simulink model "walkingRobot_stable"  (R2020a)
settings: Solver=ode15s  StartTime=0.0  StopTime=10  EnableMultiTasking=on
PreLoadFcn:
  | robotParameters
  | load('defaultsimulationinputs.mat')
values from neighbouring files (symbols this model uses):
  init_angs_L = zeros(6,1)    [robotParameters.m]
  init_angs_R = zeros(6,1)    [robotParameters.m]
  motion_time_constant = 0.001    [robotParameters.m]
libraries: simulink_extras x12, walkingRobotUtils x3, simulink x1
settings Model: SimulationMode=accelerator  Creator=bkim  LastModifiedBy=nikhil
settings DataIOCC: ReturnWorkspaceOutputs=off  OutputSaveName=simout  OutputTimes=0:0.01:10
settings OptimizationCC: LifeSpan=inf
settings DebuggingCC: AllowSymbolicDim=off  PregeneratedLibrarySubsystemCodeDiagnostic=none  SFUnexpectedBacktrackingDiag=warning  SFNoUnconditionalDefaultTransitionDiag=warning  SFExecutionAtInitializationDiag=none  UnitsInconsistencyMsg=none  ArithmeticOperatorsInVariantConditions=warning
settings SFSimCC: SimUseLocalCustomCode=off  CustomCodeUndefinedFunction=UseInterfaceOnly
settings RTWCC: RTWUseLocalCustomCode=off
settings CodeAppCC: StateflowObjectComments=on
settings GRTTargetCC: TargetLangStandard=C89/C90 (ANSI)
settings ConfigComp: CovMetricSettings=dw  CovHtmlReporting=on  CovSaveCumulativeToWorkspaceVar=on  CovSaveSingleToWorkspaceVar=on  CovExternalEMLEnable=off  CovSFcnEnable=off
settings SimscapeCC: SimscapeNormalizeSystem=off  SimscapeLogOpenViewer=on  SimscapeLogLimitData=off  SimscapeLogDataHistory=10000
settings ConfigurationSet: Description=SimMechanics 2G
settings DiagnosticsConfigSet: SimMechanicsRigidlyBoundBlock=none
settings ExplorerConfigSet: InternalSimMechanicsExplorerSettings="<ExplorerConfiguration><canonicalview>default</canonicalview><AnimationSetting><BasePlaybackSpeed>1.0</BasePlaybackSpeed><PlaybackSpeedFactor>1.0</PlaybackSpeedFactor></AnimationSetting><TilePanel><TileInfo><Tiles Columns=\"1\" Count=\"1\" Rows=\"1\"><Column Weight=\"1\"/><Row Weight=\"1\"/><Tile Height=\"1\" Width=\"1\" X=\"0\" Y=\"0\"/></Tiles></TileInfo><SceneInfo><SceneViewer><BGColor><R>0.60000002384185791</R><G>0.60000002384185791</G><B>0.60000002384185791</B></BGColor><Camera><DoPerspective>off</DoPerspective><Position><X>-7.90762128242833562</X><Y>23.8081096481694914</Y><Z>5.91146841204722939</Z></Position><Center><X>-0.406277996262525587</X><Y>0.615564294304502546</Y><Z>-0.277309600720595628</Z></Center><Up><X>0.182671955115720652</X><Y>-0.197900690545468771</Y><Z>0.963050504125213092</Z></Up><ViewLimDist>1</ViewLimDist><YLim>2.56954837368236522</YLim><XLim>3.29520786810192234</XLim></Camera></SceneViewer></SceneInfo></TilePanel><MechEditorPanel><Cameras/><GfxPanelCameraMap/><VideoCreator><PlaybackSpeedRatio>1.0</PlaybackSpeedRatio><FrameRate>30</FrameRate><VideoFormat>Motion JPEG AVI</VideoFormat><FrameSize>auto</FrameSize></VideoCreator></MechEditorPanel></ExplorerConfiguration>"

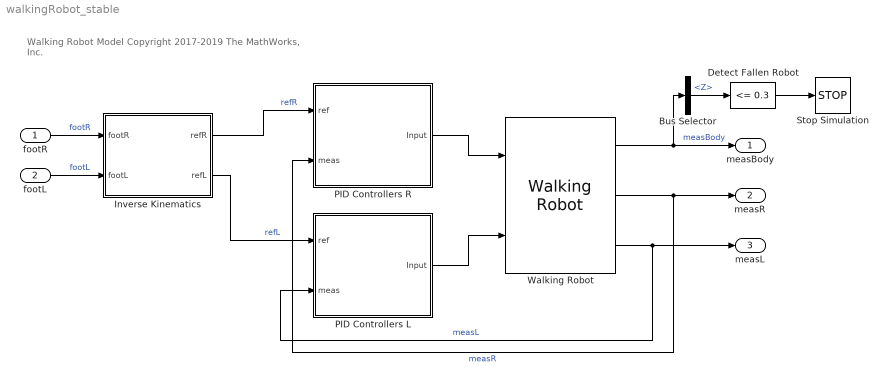
== system walkingRobot_stable ==
  note: Walking Robot Model
      |
      | Copyright 2017-2019 The MathWorks, Inc.
  footR : Inport
  footL : Inport  Port=2
  Bus Selector : BusSelector  OutputSignals=Z
  Detect Fallen Robot : simulink/Logic and Bit Operations/Compare To Constant  relop=<=  const=0.3  OutDataTypeStr=boolean
  Inverse Kinematics : Subsystem
  PID Controllers L : Subsystem
  PID Controllers R : Subsystem
  Stop Simulation : Stop
  Walking Robot : walkingRobotUtils/Walking Robot  SystemSampleTime=-1  Latency=0  AutoFrameSizeCalculation=off
  measBody : Outport  VectorParamsAs1DForOutWhenUnconnected=off
  measR : Outport  Port=2  VectorParamsAs1DForOutWhenUnconnected=off
  measL : Outport  Port=3  VectorParamsAs1DForOutWhenUnconnected=off
  wires:
  Walking Robot/3 -> PID Controllers L/2(meas), measL/1  "measL"
  Walking Robot/2 -> PID Controllers R/2(meas), measR/1  "measR"
  PID Controllers R/1(Input) -> Walking Robot/1
  PID Controllers L/1(Input) -> Walking Robot/2
  footR/1 -> Inverse Kinematics/1(footR)  "footR"
  footL/1 -> Inverse Kinematics/2(footL)  "footL"
  Walking Robot/1 -> Bus Selector/1, measBody/1  "measBody"
  Bus Selector/1 -> Detect Fallen Robot/1  "<Z>"
  Detect Fallen Robot/1 -> Stop Simulation/1
  Inverse Kinematics/1(refR) -> PID Controllers R/1(ref)  "refR"
  Inverse Kinematics/2(refL) -> PID Controllers L/1(ref)  "refL"

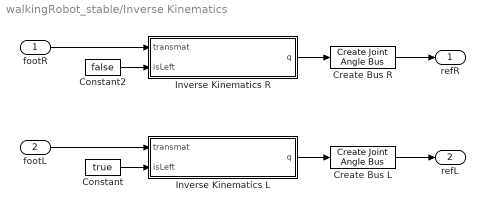
== system walkingRobot_stable/Inverse Kinematics ==
  footR : Inport
  footL : Inport  Port=2
  Constant : Constant  Value=true
  Constant2 : Constant  Value=false
  Create Bus L : walkingRobotUtils/Create Joint Angle Bus  SystemSampleTime=-1  Latency=0  AutoFrameSizeCalculation=off
  Create Bus R : walkingRobotUtils/Create Joint Angle Bus  SystemSampleTime=-1  Latency=0  AutoFrameSizeCalculation=off
  Inverse Kinematics L : MATLAB Function  TreatAsAtomicUnit=on
  Inverse Kinematics R : MATLAB Function  TreatAsAtomicUnit=on
  refR : Outport
  refL : Outport  Port=2
  wires:
  footR/1 -> Inverse Kinematics R/1(transmat)
  Inverse Kinematics L/1(q) -> Create Bus L/1
  Constant2/1 -> Inverse Kinematics R/2(isLeft)
  Create Bus R/1 -> refR/1
  Create Bus L/1 -> refL/1
  Constant/1 -> Inverse Kinematics L/2(isLeft)
  Inverse Kinematics R/1(q) -> Create Bus R/1
  footL/1 -> Inverse Kinematics L/1(transmat)

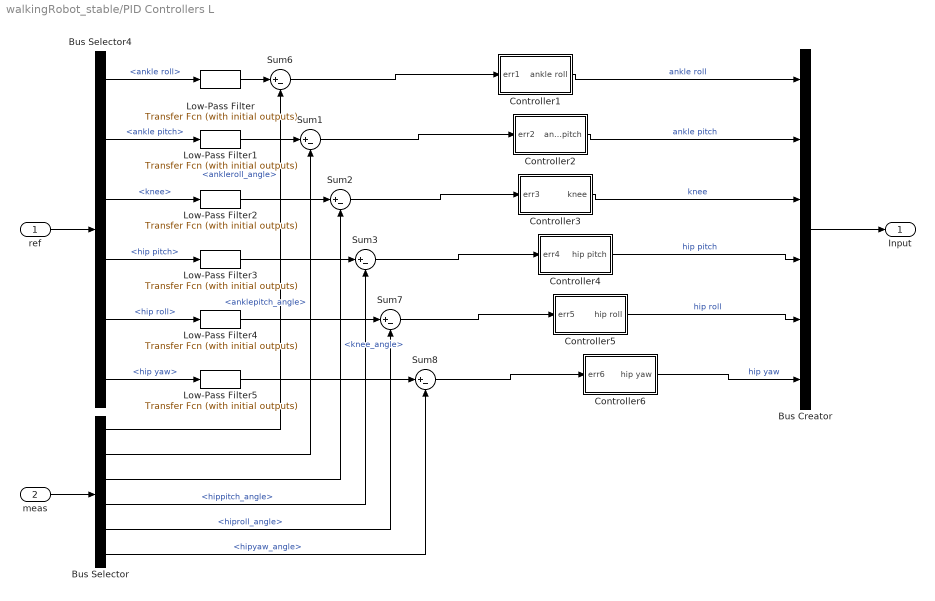
== system walkingRobot_stable/PID Controllers L ==
  ref : Inport
  meas : Inport  Port=2
  Bus Creator : BusCreator  Inputs=6
  Bus Selector : BusSelector  OutputSignals=ankleroll_angle,anklepitch_angle,knee_angle,hippitch_angle,hiproll_angle,hipyaw_angle
  Bus Selector4 : BusSelector  OutputSignals=ankle roll,ankle pitch,knee,hip pitch,hip roll,hip yaw
  Controller1 : Subsystem
  Controller2 : Subsystem
  Controller3 : Subsystem
  Controller4 : Subsystem
  Controller5 : Subsystem
  Controller6 : Subsystem
  Low-Pass Filter : simulink_extras/Additional Linear/Transfer Fcn (with initial outputs)  N=[(1/motion_time_constant)^2]  D=[1 2/motion_time_constant (1/motion_time_constant)^2]  Y0=init_angs_L(6)  U0=init_angs_L(6)
  Low-Pass Filter1 : simulink_extras/Additional Linear/Transfer Fcn (with initial outputs)  N=[(1/motion_time_constant)^2]  D=[1 2/motion_time_constant (1/motion_time_constant)^2]  Y0=init_angs_L(5)  U0=init_angs_L(5)
  Low-Pass Filter2 : simulink_extras/Additional Linear/Transfer Fcn (with initial outputs)  N=[(1/motion_time_constant)^2]  D=[1 2/motion_time_constant (1/motion_time_constant)^2]  Y0=init_angs_L(4)  U0=init_angs_L(4)
  Low-Pass Filter3 : simulink_extras/Additional Linear/Transfer Fcn (with initial outputs)  N=[(1/motion_time_constant)^2]  D=[1 2/motion_time_constant (1/motion_time_constant)^2]  Y0=init_angs_L(3)  U0=init_angs_L(3)
  Low-Pass Filter4 : simulink_extras/Additional Linear/Transfer Fcn (with initial outputs)  N=[(1/motion_time_constant)^2]  D=[1 2/motion_time_constant (1/motion_time_constant)^2]  Y0=init_angs_L(2)  U0=init_angs_L(2)
  Low-Pass Filter5 : simulink_extras/Additional Linear/Transfer Fcn (with initial outputs)  N=[(1/motion_time_constant)^2]  D=[1 2/motion_time_constant (1/motion_time_constant)^2]  Y0=init_angs_L(1)  U0=init_angs_L(1)
  Sum{1..3,6..8} (6 alike) : Sum  Inputs=|+-
  Input : Outport  VectorParamsAs1DForOutWhenUnconnected=off
  wires:
  Low-Pass Filter5/1 -> Sum8/1
  Low-Pass Filter/1 -> Sum6/1
  Bus Selector4/6 -> Low-Pass Filter5/1  "<hip yaw>"
  Bus Selector4/2 -> Low-Pass Filter1/1  "<ankle pitch>"
  Bus Selector4/4 -> Low-Pass Filter3/1  "<hip pitch>"
  Controller6/1(hip yaw) -> Bus Creator/6  "hip yaw"
  Bus Selector4/3 -> Low-Pass Filter2/1  "<knee>"
  Bus Selector4/1 -> Low-Pass Filter/1  "<ankle roll>"
  Bus Selector/3 -> Sum2/2  "<knee_angle>"
  Bus Selector4/5 -> Low-Pass Filter4/1  "<hip roll>"
  ref/1 -> Bus Selector4/1
  Low-Pass Filter3/1 -> Sum3/1
  Bus Selector/6 -> Sum8/2  "<hipyaw_angle>"
  Bus Selector/5 -> Sum7/2  "<hiproll_angle>"
  Low-Pass Filter1/1 -> Sum1/1
  Bus Creator/1 -> Input/1
  Bus Selector/1 -> Sum6/2  "<ankleroll_angle>"
  Low-Pass Filter2/1 -> Sum2/1
  Low-Pass Filter4/1 -> Sum7/1
  Bus Selector/4 -> Sum3/2  "<hippitch_angle>"
  Bus Selector/2 -> Sum1/2  "<anklepitch_angle>"
  meas/1 -> Bus Selector/1
  Controller1/1(ankle roll) -> Bus Creator/1  "ankle roll"
  Sum7/1 -> Controller5/1(err5)
  Sum6/1 -> Controller1/1(err1)
  Controller3/1(knee) -> Bus Creator/3  "knee"
  Sum1/1 -> Controller2/1(err2)
  Controller4/1(hip pitch) -> Bus Creator/4  "hip pitch"
  Sum2/1 -> Controller3/1(err3)
  Sum8/1 -> Controller6/1(err6)
  Sum3/1 -> Controller4/1(err4)
  Controller5/1(hip roll) -> Bus Creator/5  "hip roll"
  Controller2/1(ankle pitch) -> Bus Creator/2  "ankle pitch"

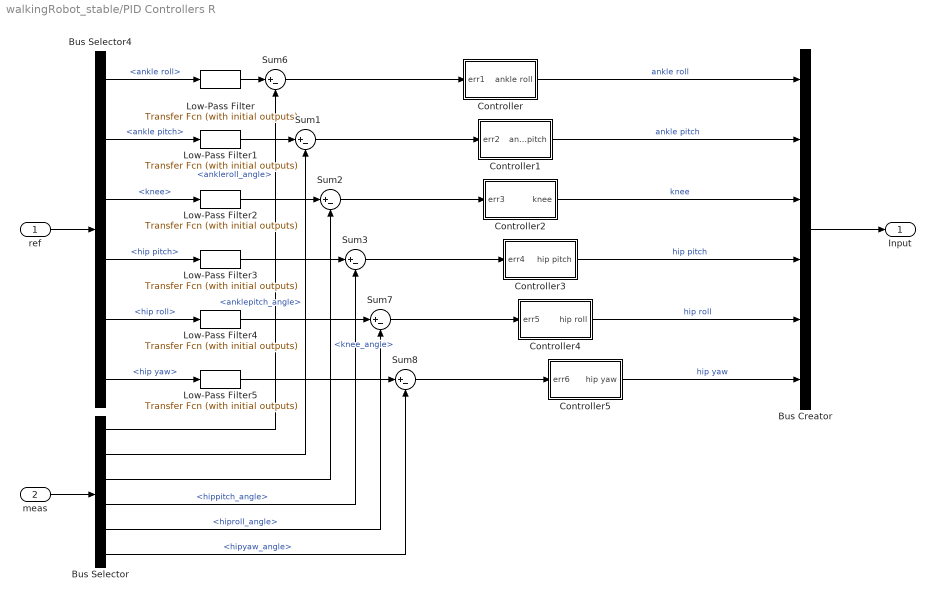
== system walkingRobot_stable/PID Controllers R ==
  ref : Inport
  meas : Inport  Port=2
  Bus Creator : BusCreator  Inputs=6
  Bus Selector : BusSelector  OutputSignals=ankleroll_angle,anklepitch_angle,knee_angle,hippitch_angle,hiproll_angle,hipyaw_angle
  Bus Selector4 : BusSelector  OutputSignals=ankle roll,ankle pitch,knee,hip pitch,hip roll,hip yaw
  Controller : Subsystem
  Controller1 : Subsystem
  Controller2 : Subsystem
  Controller3 : Subsystem
  Controller4 : Subsystem
  Controller5 : Subsystem
  Low-Pass Filter : simulink_extras/Additional Linear/Transfer Fcn (with initial outputs)  N=[(1/motion_time_constant)^2]  D=[1 2/motion_time_constant (1/motion_time_constant)^2]  Y0=init_angs_R(6)  U0=init_angs_R(6)
  Low-Pass Filter1 : simulink_extras/Additional Linear/Transfer Fcn (with initial outputs)  N=[(1/motion_time_constant)^2]  D=[1 2/motion_time_constant (1/motion_time_constant)^2]  Y0=init_angs_R(5)  U0=init_angs_R(5)
  Low-Pass Filter2 : simulink_extras/Additional Linear/Transfer Fcn (with initial outputs)  N=[(1/motion_time_constant)^2]  D=[1 2/motion_time_constant (1/motion_time_constant)^2]  Y0=init_angs_R(4)  U0=init_angs_R(4)
  Low-Pass Filter3 : simulink_extras/Additional Linear/Transfer Fcn (with initial outputs)  N=[(1/motion_time_constant)^2]  D=[1 2/motion_time_constant (1/motion_time_constant)^2]  Y0=init_angs_R(3)  U0=init_angs_R(3)
  Low-Pass Filter4 : simulink_extras/Additional Linear/Transfer Fcn (with initial outputs)  N=[(1/motion_time_constant)^2]  D=[1 2/motion_time_constant (1/motion_time_constant)^2]  Y0=init_angs_R(2)  U0=init_angs_R(2)
  Low-Pass Filter5 : simulink_extras/Additional Linear/Transfer Fcn (with initial outputs)  N=[(1/motion_time_constant)^2]  D=[1 2/motion_time_constant (1/motion_time_constant)^2]  Y0=init_angs_R(1)  U0=init_angs_R(1)
  Sum{1..3,6..8} (6 alike) : Sum  Inputs=|+-
  Input : Outport  VectorParamsAs1DForOutWhenUnconnected=off
  wires:
  meas/1 -> Bus Selector/1
  Bus Selector/2 -> Sum1/2  "<anklepitch_angle>"
  Bus Selector/4 -> Sum3/2  "<hippitch_angle>"
  Low-Pass Filter4/1 -> Sum7/1
  Low-Pass Filter2/1 -> Sum2/1
  Sum8/1 -> Controller5/1(err6)
  Bus Selector/1 -> Sum6/2  "<ankleroll_angle>"
  Bus Creator/1 -> Input/1
  Low-Pass Filter1/1 -> Sum1/1
  Bus Selector/5 -> Sum7/2  "<hiproll_angle>"
  Controller3/1(hip pitch) -> Bus Creator/4  "hip pitch"
  Bus Selector/6 -> Sum8/2  "<hipyaw_angle>"
  Low-Pass Filter3/1 -> Sum3/1
  Controller/1(ankle roll) -> Bus Creator/1  "ankle roll"
  Sum1/1 -> Controller1/1(err2)
  Sum2/1 -> Controller2/1(err3)
  ref/1 -> Bus Selector4/1
  Sum3/1 -> Controller3/1(err4)
  Bus Selector4/5 -> Low-Pass Filter4/1  "<hip roll>"
  Sum7/1 -> Controller4/1(err5)
  Bus Selector/3 -> Sum2/2  "<knee_angle>"
  Sum6/1 -> Controller/1(err1)
  Bus Selector4/1 -> Low-Pass Filter/1  "<ankle roll>"
  Bus Selector4/3 -> Low-Pass Filter2/1  "<knee>"
  Controller2/1(knee) -> Bus Creator/3  "knee"
  Controller5/1(hip yaw) -> Bus Creator/6  "hip yaw"
  Controller1/1(ankle pitch) -> Bus Creator/2  "ankle pitch"
  Bus Selector4/4 -> Low-Pass Filter3/1  "<hip pitch>"
  Bus Selector4/2 -> Low-Pass Filter1/1  "<ankle pitch>"
  Controller4/1(hip roll) -> Bus Creator/5  "hip roll"
  Bus Selector4/6 -> Low-Pass Filter5/1  "<hip yaw>"
  Low-Pass Filter/1 -> Sum6/1
  Low-Pass Filter5/1 -> Sum8/1

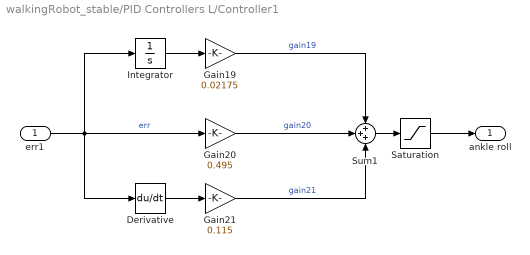
== system walkingRobot_stable/PID Controllers L/Controller1 ==
  err1 : Inport
  Derivative : Derivative
  Gain19 : Gain  Gain=0.02175
  Gain20 : Gain  Gain=0.495
  Gain21 : Gain  Gain=0.115
  Integrator : Integrator
  Saturation : Saturate  UpperLimit=15  LowerLimit=-15
  Sum1 : Sum  Inputs=+++
  ankle roll : Outport
  wires:
  Gain19/1 -> Sum1/1  "gain19"
  Saturation/1 -> ankle roll/1
  Gain20/1 -> Sum1/2  "gain20"
  Gain21/1 -> Sum1/3  "gain21"
  err1/1 -> Derivative/1, Gain20/1, Integrator/1  "err"
  Derivative/1 -> Gain21/1
  Sum1/1 -> Saturation/1
  Integrator/1 -> Gain19/1

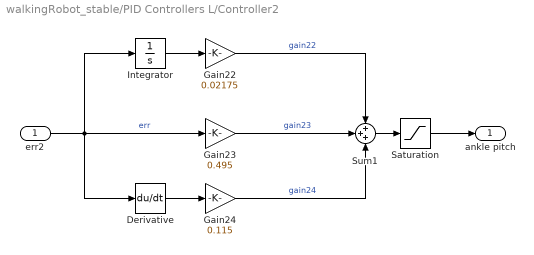
== system walkingRobot_stable/PID Controllers L/Controller2 ==
  err2 : Inport
  Derivative : Derivative
  Gain22 : Gain  Gain=0.02175
  Gain23 : Gain  Gain=0.495
  Gain24 : Gain  Gain=0.115
  Integrator : Integrator
  Saturation : Saturate  UpperLimit=15  LowerLimit=-15
  Sum1 : Sum  Inputs=+++
  ankle pitch : Outport
  wires:
  Gain22/1 -> Sum1/1  "gain22"
  Saturation/1 -> ankle pitch/1
  Gain23/1 -> Sum1/2  "gain23"
  Gain24/1 -> Sum1/3  "gain24"
  err2/1 -> Derivative/1, Gain23/1, Integrator/1  "err"
  Derivative/1 -> Gain24/1
  Sum1/1 -> Saturation/1
  Integrator/1 -> Gain22/1

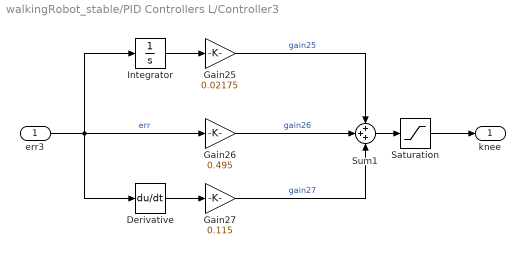
== system walkingRobot_stable/PID Controllers L/Controller3 ==
  err3 : Inport
  Derivative : Derivative
  Gain25 : Gain  Gain=0.02175
  Gain26 : Gain  Gain=0.495
  Gain27 : Gain  Gain=0.115
  Integrator : Integrator
  Saturation : Saturate  UpperLimit=15  LowerLimit=-15
  Sum1 : Sum  Inputs=+++
  knee : Outport
  wires:
  Gain25/1 -> Sum1/1  "gain25"
  Saturation/1 -> knee/1
  Gain26/1 -> Sum1/2  "gain26"
  Gain27/1 -> Sum1/3  "gain27"
  err3/1 -> Derivative/1, Gain26/1, Integrator/1  "err"
  Derivative/1 -> Gain27/1
  Sum1/1 -> Saturation/1
  Integrator/1 -> Gain25/1

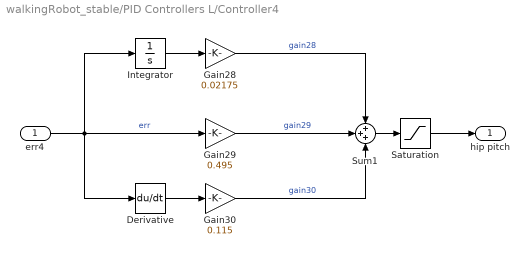
== system walkingRobot_stable/PID Controllers L/Controller4 ==
  err4 : Inport
  Derivative : Derivative
  Gain28 : Gain  Gain=0.02175
  Gain29 : Gain  Gain=0.495
  Gain30 : Gain  Gain=0.115
  Integrator : Integrator
  Saturation : Saturate  UpperLimit=15  LowerLimit=-15
  Sum1 : Sum  Inputs=+++
  hip pitch : Outport
  wires:
  Gain28/1 -> Sum1/1  "gain28"
  Saturation/1 -> hip pitch/1
  Gain29/1 -> Sum1/2  "gain29"
  Gain30/1 -> Sum1/3  "gain30"
  err4/1 -> Derivative/1, Gain29/1, Integrator/1  "err"
  Derivative/1 -> Gain30/1
  Sum1/1 -> Saturation/1
  Integrator/1 -> Gain28/1

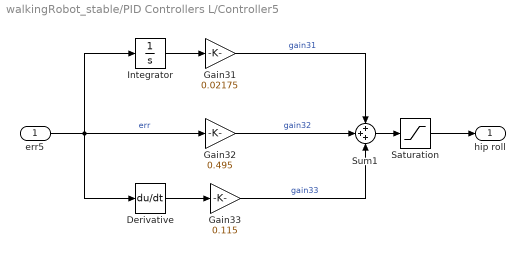
== system walkingRobot_stable/PID Controllers L/Controller5 ==
  err5 : Inport
  Derivative : Derivative
  Gain31 : Gain  Gain=0.02175
  Gain32 : Gain  Gain=0.495
  Gain33 : Gain  Gain=0.115
  Integrator : Integrator
  Saturation : Saturate  UpperLimit=15  LowerLimit=-15
  Sum1 : Sum  Inputs=+++
  hip roll : Outport
  wires:
  Gain31/1 -> Sum1/1  "gain31"
  Saturation/1 -> hip roll/1
  Gain32/1 -> Sum1/2  "gain32"
  Gain33/1 -> Sum1/3  "gain33"
  err5/1 -> Derivative/1, Gain32/1, Integrator/1  "err"
  Derivative/1 -> Gain33/1
  Sum1/1 -> Saturation/1
  Integrator/1 -> Gain31/1

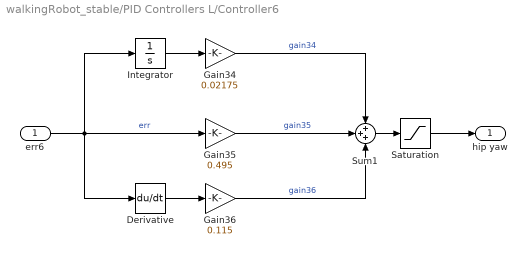
== system walkingRobot_stable/PID Controllers L/Controller6 ==
  err6 : Inport
  Derivative : Derivative
  Gain34 : Gain  Gain=0.02175
  Gain35 : Gain  Gain=0.495
  Gain36 : Gain  Gain=0.115
  Integrator : Integrator
  Saturation : Saturate  UpperLimit=15  LowerLimit=-15
  Sum1 : Sum  Inputs=+++
  hip yaw : Outport
  wires:
  Gain34/1 -> Sum1/1  "gain34"
  Saturation/1 -> hip yaw/1
  Gain35/1 -> Sum1/2  "gain35"
  Gain36/1 -> Sum1/3  "gain36"
  err6/1 -> Derivative/1, Gain35/1, Integrator/1  "err"
  Derivative/1 -> Gain36/1
  Sum1/1 -> Saturation/1
  Integrator/1 -> Gain34/1

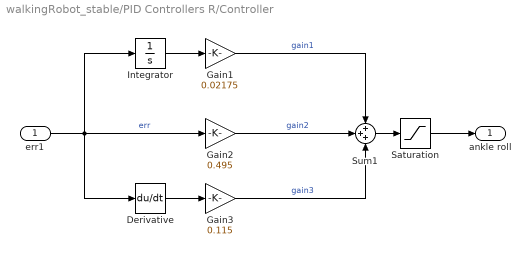
== system walkingRobot_stable/PID Controllers R/Controller ==
  err1 : Inport
  Derivative : Derivative
  Gain1 : Gain  Gain=0.02175
  Gain2 : Gain  Gain=0.495
  Gain3 : Gain  Gain=0.115
  Integrator : Integrator
  Saturation : Saturate  UpperLimit=15  LowerLimit=-15
  Sum1 : Sum  Inputs=+++
  ankle roll : Outport
  wires:
  Gain1/1 -> Sum1/1  "gain1"
  Saturation/1 -> ankle roll/1
  Gain2/1 -> Sum1/2  "gain2"
  Gain3/1 -> Sum1/3  "gain3"
  err1/1 -> Derivative/1, Gain2/1, Integrator/1  "err"
  Derivative/1 -> Gain3/1
  Sum1/1 -> Saturation/1
  Integrator/1 -> Gain1/1

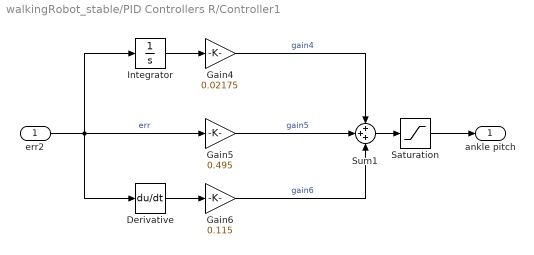
== system walkingRobot_stable/PID Controllers R/Controller1 ==
  err2 : Inport
  Derivative : Derivative
  Gain4 : Gain  Gain=0.02175
  Gain5 : Gain  Gain=0.495
  Gain6 : Gain  Gain=0.115
  Integrator : Integrator
  Saturation : Saturate  UpperLimit=15  LowerLimit=-15
  Sum1 : Sum  Inputs=+++
  ankle pitch : Outport
  wires:
  Gain4/1 -> Sum1/1  "gain4"
  Saturation/1 -> ankle pitch/1
  Gain5/1 -> Sum1/2  "gain5"
  Gain6/1 -> Sum1/3  "gain6"
  err2/1 -> Derivative/1, Gain5/1, Integrator/1  "err"
  Derivative/1 -> Gain6/1
  Sum1/1 -> Saturation/1
  Integrator/1 -> Gain4/1

== system walkingRobot_stable/PID Controllers R/Controller2 ==
  err3 : Inport
  Derivative : Derivative
  Gain7 : Gain  Gain=0.02175
  Gain8 : Gain  Gain=0.495
  Gain9 : Gain  Gain=0.115
  Integrator : Integrator
  Saturation : Saturate  UpperLimit=15  LowerLimit=-15
  Sum1 : Sum  Inputs=+++
  knee : Outport
  wires:
  Gain7/1 -> Sum1/1  "gain7"
  Saturation/1 -> knee/1
  Gain8/1 -> Sum1/2  "gain8"
  Gain9/1 -> Sum1/3  "gain9"
  err3/1 -> Derivative/1, Gain8/1, Integrator/1  "err"
  Derivative/1 -> Gain9/1
  Sum1/1 -> Saturation/1
  Integrator/1 -> Gain7/1

== system walkingRobot_stable/PID Controllers R/Controller3 ==
  err4 : Inport
  Derivative : Derivative
  Gain10 : Gain  Gain=0.02175
  Gain11 : Gain  Gain=0.495
  Gain12 : Gain  Gain=0.115
  Integrator : Integrator
  Saturation : Saturate  UpperLimit=15  LowerLimit=-15
  Sum1 : Sum  Inputs=+++
  hip pitch : Outport
  wires:
  Gain10/1 -> Sum1/1  "gain10"
  Saturation/1 -> hip pitch/1
  Gain11/1 -> Sum1/2  "gain11"
  Gain12/1 -> Sum1/3  "gain12"
  err4/1 -> Derivative/1, Gain11/1, Integrator/1  "err"
  Derivative/1 -> Gain12/1
  Sum1/1 -> Saturation/1
  Integrator/1 -> Gain10/1

== system walkingRobot_stable/PID Controllers R/Controller4 ==
  err5 : Inport
  Derivative : Derivative
  Gain13 : Gain  Gain=0.02175
  Gain14 : Gain  Gain=0.495
  Gain15 : Gain  Gain=0.115
  Integrator : Integrator
  Saturation : Saturate  UpperLimit=15  LowerLimit=-15
  Sum1 : Sum  Inputs=+++
  hip roll : Outport
  wires:
  Gain13/1 -> Sum1/1  "gain13"
  Saturation/1 -> hip roll/1
  Gain14/1 -> Sum1/2  "gain14"
  Gain15/1 -> Sum1/3  "gain15"
  err5/1 -> Derivative/1, Gain14/1, Integrator/1  "err"
  Derivative/1 -> Gain15/1
  Sum1/1 -> Saturation/1
  Integrator/1 -> Gain13/1

== system walkingRobot_stable/PID Controllers R/Controller5 ==
  err6 : Inport
  Derivative : Derivative
  Gain16 : Gain  Gain=0.02175
  Gain17 : Gain  Gain=0.495
  Gain18 : Gain  Gain=0.115
  Integrator : Integrator
  Saturation : Saturate  UpperLimit=15  LowerLimit=-15
  Sum1 : Sum  Inputs=+++
  hip yaw : Outport
  wires:
  Gain16/1 -> Sum1/1  "gain16"
  Saturation/1 -> hip yaw/1
  Gain17/1 -> Sum1/2  "gain17"
  Gain18/1 -> Sum1/3  "gain18"
  err6/1 -> Derivative/1, Gain17/1, Integrator/1  "err"
  Derivative/1 -> Gain18/1
  Sum1/1 -> Saturation/1
  Integrator/1 -> Gain16/1

== matlab function walkingRobot_stable/Inverse Kinematics/Inverse Kinematics R ==
  data: transmat input; q output; isLeft input
function q = inverseKinematics(transmat, isLeft)
q = invKinBody2Foot(transmat, isLeft);

== matlab function walkingRobot_stable/Inverse Kinematics/Inverse Kinematics L ==
  data: transmat input; q output; isLeft input
function q = inverseKinematics(transmat, isLeft)
q = invKinBody2Foot(transmat, isLeft);
